simulink model "Model_Main_v4"  (R2025a)
settings: Solver=VariableStepAuto  StartTime=0.0  StopTime=10.0  RelTol=1e-3  AbsTol=1e-3
undefined symbols (not defined in the file): area_air, cp_air, eta_map, HC_min, HC_nom, rho_air, speed_bp_rpm, torque_bp_Nm, vel_air_nom
libraries: fl_lib x26, nesl_utility x14, SimscapeFluids_lib x5
(part 3 of 3)

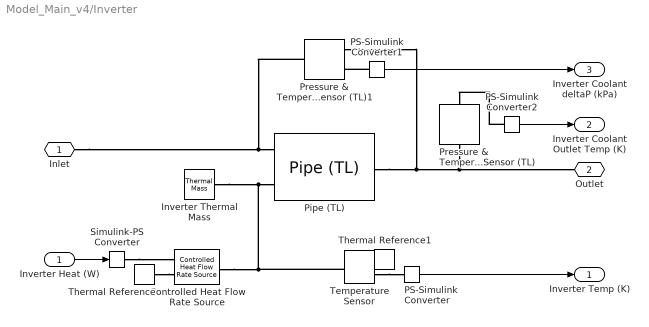
== system Model_Main_v4/Inverter ==
  Inverter Heat (W) : Inport
  Controlled Heat Flow Rate Source : fl_lib/Thermal/Thermal Sources/Controlled Heat Flow Rate Source
  Inverter Thermal Mass : fl_lib/Thermal/Thermal Elements/Thermal Mass  mass_type=foundation.enum.constant_variable.constant  mass=10 kg  sp_heat=900 J/(K*kg)  mass_min=1e-6 kg  num_ports=foundation.enum.numPorts2.one  m_specify=off  m_priority=High  m=1 kg  m_nominal_specify=off  m_nominal_value=1  m_nominal_unit=kg  T_specify=off  T_priority=High  T=300 K  T_nominal_specify=off  T_nominal_value=1  T_nominal_unit=K  Q_specify=off  Q_priority=None  Q=0 W  Q_nominal_specify=off  Q_nominal_value=1  Q_nominal_unit=W
  PS-Simulink Converter : nesl_utility/PS-Simulink Converter  PhysicalDomain=network_engine_domain  SubClassName=ps_output  LeftPortType=input  RightPortType=output  PseudoPeriodic=off  Frequencies=[]  VectorFormat=inherit  Unit=degC  AffineConversion=off
  PS-Simulink Converter1 : nesl_utility/PS-Simulink Converter  PhysicalDomain=network_engine_domain  SubClassName=ps_output  LeftPortType=input  RightPortType=output  PseudoPeriodic=off  Frequencies=[]  VectorFormat=inherit  Unit=kPa  AffineConversion=off
  PS-Simulink Converter2 : nesl_utility/PS-Simulink Converter  PhysicalDomain=network_engine_domain  SubClassName=ps_output  LeftPortType=input  RightPortType=output  PseudoPeriodic=off  Frequencies=[]  VectorFormat=inherit  Unit=degC  AffineConversion=off
  Pipe (TL) : fl_lib/Thermal Liquid/Elements/Pipe (TL)  length=3 m  area=5e-5 m^2  Dh=0.007 m  length_add=1 m  roughness=15e-6 m  Re_lam=2000  Re_tur=4000  shape_factor=64  Nu_lam=3.66  dynamic_compressibility=true  inertia=false  p0=0.101325 MPa  T0=293.15 K  mdot0=0 kg/s  p_nominal=0.101325 MPa  T_nominal=293.15 K
  Pressure & Temperature Sensor (TL) : fl_lib/Thermal Liquid/Sensors/Pressure & Temperature Sensor (TL)  reference=foundation.enum.MeasurementReference.absolute  pressure=false  pressure_spec=foundation.enum.PressureMeasementSpec.Absolute  temperature=true
      settings: InternalSimscapePortConfiguration="{\"Bottom\":[{\"id\":\"T\",\"label\":\"T\",\"type\":\"output\"}],\"Left\":[{\"id\":\"A\",\"label\":\"A\",\"type\":\"foundation.thermal_liquid.thermal_liquid\"}],\"Right\":[],\"Top\":[]}"
  Pressure & Temperature Sensor (TL)1 : fl_lib/Thermal Liquid/Sensors/Pressure & Temperature Sensor (TL)  reference=foundation.enum.MeasurementReference.difference  pressure=true  pressure_spec=foundation.enum.PressureMeasementSpec.Absolute  temperature=false
      settings: InternalSimscapePortConfiguration="{\"Bottom\":[],\"Left\":[{\"id\":\"A\",\"label\":\"A\",\"type\":\"foundation.thermal_liquid.thermal_liquid\"}],\"Right\":[{\"id\":\"B\",\"label\":\"B\",\"type\":\"foundation.thermal_liquid.thermal_liquid\"},{\"id\":\"P\",\"label\":\"P\",\"type\":\"output\"}],\"Top\":[]}"
  Simulink-PS Converter : nesl_utility/Simulink-PS Converter  PhysicalDomain=network_engine_domain  SubClassName=ps_input  LeftPortType=input  RightPortType=output  PseudoPeriodic=off  Frequencies=[]  NoiseDistribution=none  NoiseParameters=[]  Unit=W  AffineConversion=off  FilteringAndDerivatives=provide  SimscapeFilterOrder=1  InputFilterTimeConstant=0.001  UdotUserProvided=0
  Temperature Sensor : fl_lib/Thermal/Thermal Sensors/Temperature Sensor  temperature_measure=foundation.enum.MeasurementReference.difference
  Thermal Reference : fl_lib/Thermal/Thermal Elements/Thermal Reference
  Thermal Reference1 : fl_lib/Thermal/Thermal Elements/Thermal Reference
  Inlet : PMIOPort  Side=Left
  Outlet : PMIOPort  Port=2  Side=Right
  Inverter Temp (K) : Outport
  Inverter Coolant Outlet Temp (K) : Outport  Port=2
  Inverter Coolant deltaP (kPa) : Outport  Port=3
  wires:
  Inverter Heat (W)/1 -> Simulink-PS Converter/1
  PS-Simulink Converter/1 -> Inverter Temp (K)/1
  PS-Simulink Converter2/1 -> Inverter Coolant Outlet Temp (K)/1
  PS-Simulink Converter1/1 -> Inverter Coolant deltaP (kPa)/1
  connections:
  Inlet/RConn1 -- Pressure & Temperature Sensor (TL)1/LConn1 -- Pipe (TL)/LConn1
  Pipe (TL)/RConn1 -- Pressure & Temperature Sensor (TL)1/RConn1 -- Pressure & Temperature Sensor (TL)/LConn1 -- Outlet/RConn1
  Inverter Thermal Mass/LConn1 -- Temperature Sensor/LConn1 -- Controlled Heat Flow Rate Source/LConn1 -- Pipe (TL)/LConn2
  Thermal Reference/LConn1 -- Controlled Heat Flow Rate Source/RConn2
  Simulink-PS Converter/RConn1 -- Controlled Heat Flow Rate Source/RConn1
  Thermal Reference1/LConn1 -- Temperature Sensor/RConn1
  Temperature Sensor/RConn2 -- PS-Simulink Converter/LConn1
  PS-Simulink Converter1/LConn1 -- Pressure & Temperature Sensor (TL)1/RConn2
  PS-Simulink Converter2/LConn1 -- Pressure & Temperature Sensor (TL)/RConn1

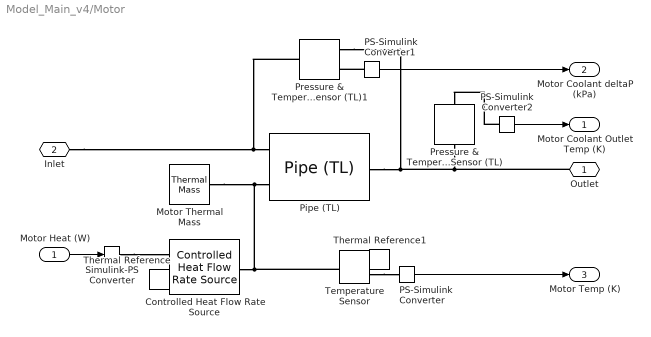
== system Model_Main_v4/Motor ==
  Motor Heat (W) : Inport
  Controlled Heat Flow Rate Source : fl_lib/Thermal/Thermal Sources/Controlled Heat Flow Rate Source
  Motor Thermal Mass : fl_lib/Thermal/Thermal Elements/Thermal Mass  mass_type=foundation.enum.constant_variable.constant  mass=24 kg  sp_heat=449 J/(K*kg)  mass_min=1e-6 kg  num_ports=foundation.enum.numPorts2.one  m_specify=off  m_priority=High  m=1 kg  m_nominal_specify=off  m_nominal_value=1  m_nominal_unit=kg  T_specify=off  T_priority=High  T=300 K  T_nominal_specify=off  T_nominal_value=1  T_nominal_unit=K  Q_specify=off  Q_priority=None  Q=0 W  Q_nominal_specify=off  Q_nominal_value=1  Q_nominal_unit=W
  PS-Simulink Converter : nesl_utility/PS-Simulink Converter  PhysicalDomain=network_engine_domain  SubClassName=ps_output  LeftPortType=input  RightPortType=output  PseudoPeriodic=off  Frequencies=[]  VectorFormat=inherit  Unit=degC  AffineConversion=off
  PS-Simulink Converter1 : nesl_utility/PS-Simulink Converter  PhysicalDomain=network_engine_domain  SubClassName=ps_output  LeftPortType=input  RightPortType=output  PseudoPeriodic=off  Frequencies=[]  VectorFormat=inherit  Unit=kPa  AffineConversion=off
  PS-Simulink Converter2 : nesl_utility/PS-Simulink Converter  PhysicalDomain=network_engine_domain  SubClassName=ps_output  LeftPortType=input  RightPortType=output  PseudoPeriodic=off  Frequencies=[]  VectorFormat=inherit  Unit=degC  AffineConversion=off
  Pipe (TL) : fl_lib/Thermal Liquid/Elements/Pipe (TL)  length=0.8 m  area=7.5e-6 m^2  Dh=0.023077 m  length_add=1 m  roughness=15e-6 m  Re_lam=2000  Re_tur=4000  shape_factor=64  Nu_lam=3.66  dynamic_compressibility=true  inertia=false  p0=0.101325 MPa  T0=293.15 K  mdot0=0 kg/s  p_nominal=0.101325 MPa  T_nominal=293.15 K
  Pressure & Temperature Sensor (TL) : fl_lib/Thermal Liquid/Sensors/Pressure & Temperature Sensor (TL)  reference=foundation.enum.MeasurementReference.absolute  pressure=false  pressure_spec=foundation.enum.PressureMeasementSpec.Absolute  temperature=true
      settings: InternalSimscapePortConfiguration="{\"Bottom\":[{\"id\":\"T\",\"label\":\"T\",\"type\":\"output\"}],\"Left\":[{\"id\":\"A\",\"label\":\"A\",\"type\":\"foundation.thermal_liquid.thermal_liquid\"}],\"Right\":[],\"Top\":[]}"
  Pressure & Temperature Sensor (TL)1 : fl_lib/Thermal Liquid/Sensors/Pressure & Temperature Sensor (TL)  reference=foundation.enum.MeasurementReference.difference  pressure=true  pressure_spec=foundation.enum.PressureMeasementSpec.Absolute  temperature=false
      settings: InternalSimscapePortConfiguration="{\"Bottom\":[],\"Left\":[{\"id\":\"A\",\"label\":\"A\",\"type\":\"foundation.thermal_liquid.thermal_liquid\"}],\"Right\":[{\"id\":\"B\",\"label\":\"B\",\"type\":\"foundation.thermal_liquid.thermal_liquid\"},{\"id\":\"P\",\"label\":\"P\",\"type\":\"output\"}],\"Top\":[]}"
  Simulink-PS Converter : nesl_utility/Simulink-PS Converter  PhysicalDomain=network_engine_domain  SubClassName=ps_input  LeftPortType=input  RightPortType=output  PseudoPeriodic=off  Frequencies=[]  NoiseDistribution=none  NoiseParameters=[]  Unit=W  AffineConversion=off  FilteringAndDerivatives=provide  SimscapeFilterOrder=1  InputFilterTimeConstant=0.001  UdotUserProvided=0
  Temperature Sensor : fl_lib/Thermal/Thermal Sensors/Temperature Sensor  temperature_measure=foundation.enum.MeasurementReference.difference
  Thermal Reference : fl_lib/Thermal/Thermal Elements/Thermal Reference
  Thermal Reference1 : fl_lib/Thermal/Thermal Elements/Thermal Reference
  Outlet : PMIOPort  Side=Left
  Inlet : PMIOPort  Port=2  Side=Right
  Motor Coolant Outlet Temp (K) : Outport
  Motor Coolant deltaP (kPa) : Outport  Port=2
  Motor Temp (K) : Outport  Port=3
  wires:
  Motor Heat (W)/1 -> Simulink-PS Converter/1
  PS-Simulink Converter/1 -> Motor Temp (K)/1
  PS-Simulink Converter2/1 -> Motor Coolant Outlet Temp (K)/1
  PS-Simulink Converter1/1 -> Motor Coolant deltaP (kPa)/1
  connections:
  Pipe (TL)/LConn1 -- Inlet/RConn1 -- Pressure & Temperature Sensor (TL)1/LConn1
  Pressure & Temperature Sensor (TL)1/RConn1 -- Pipe (TL)/RConn1 -- Pressure & Temperature Sensor (TL)/LConn1 -- Outlet/RConn1
  Motor Thermal Mass/LConn1 -- Temperature Sensor/LConn1 -- Controlled Heat Flow Rate Source/LConn1 -- Pipe (TL)/LConn2
  Thermal Reference/LConn1 -- Controlled Heat Flow Rate Source/RConn2
  Simulink-PS Converter/RConn1 -- Controlled Heat Flow Rate Source/RConn1
  Thermal Reference1/LConn1 -- Temperature Sensor/RConn1
  Temperature Sensor/RConn2 -- PS-Simulink Converter/LConn1
  PS-Simulink Converter1/LConn1 -- Pressure & Temperature Sensor (TL)1/RConn2
  PS-Simulink Converter2/LConn1 -- Pressure & Temperature Sensor (TL)/RConn1

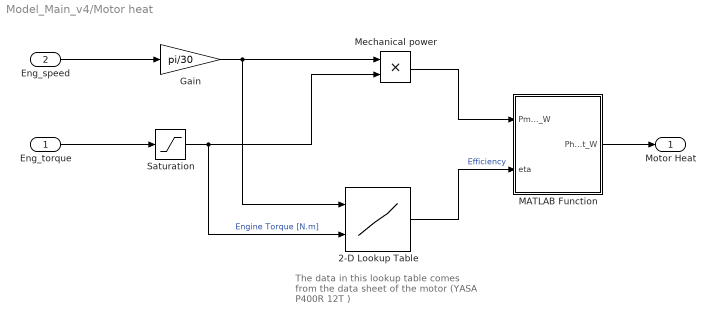
== system Model_Main_v4/Motor heat ==
  note: The data in this lookup table comes from the data sheet of the motor (YASA P400R 12T )
  Eng_torque : Inport
  Eng_speed : Inport  Port=2
  2-D Lookup Table : Lookup_n-D  BreakpointsForDimension1=torque_bp_Nm  BreakpointsForDimension2=speed_bp_rpm  Table=eta_map  InternalRulePriority=Speed  RndMeth=Simplest
      settings: InputPortMap=u0,u1
  Gain : Gain  Gain=pi/30
  MATLAB Function : MATLAB Function  TreatAsAtomicUnit=on
  Mechanical power : Product
  Saturation : Saturate  UpperLimit=inf  LowerLimit=0
  Motor Heat : Outport  VectorParamsAs1DForOutWhenUnconnected=off
  wires:
  Saturation/1 -> 2-D Lookup Table/2, Mechanical power/2  "Engine Torque [N.m]"
  Eng_torque/1 -> Saturation/1
  Gain/1 -> 2-D Lookup Table/1, Mechanical power/1
  Eng_speed/1 -> Gain/1
  2-D Lookup Table/1 -> MATLAB Function/2(eta)  "Efficiency"
  Mechanical power/1 -> MATLAB Function/1(Pmech_W)
  MATLAB Function/1(Pheat_W) -> Motor Heat/1

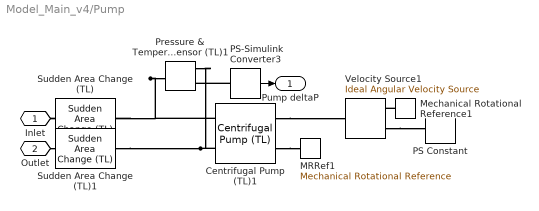
== system Model_Main_v4/Pump ==
  Centrifugal Pump (TL)1 : SimscapeFluids_lib/Thermal Liquid/Pumps & Motors/Centrifugal Pump (TL)  pump_parameterization=fluids.thermal_liquid.pumps_motors.enum.CentrifugalPumpParameterization.Table1D  capacity_ref_nominal=45 lpm  head_ref_nominal=40 m  power_ref_nominal=0.85 kW  head_ref_max=60 m  capacity_ref_max=80 lpm  omega_ref_analytic=1770 rpm  flow_rate_1D_TLU=|  head_1D_TLU=|  power_1D_TLU=[37 : 0.55 : 53]' kW  omega_ref_1D=3500 rpm  rho_ref_1D=820 kg/m^3  omega_threshold_factor=1e-2  flow_rate_2D_TLU=[16.67, 23.33, 30, 40, 53.33, 60] lpm  omega_2D_TLU=[2450, 2800, 3150, 3500] rpm  head_2D_TLU=[25, 32.7, 42.5, 50; 24, 31.7, 41, 49; 22.7, 30.5, 39, 47.5; 20, 28, 36, 45; 15.7, 24, 32, 40; 12.5, 21, 29.5, 37.5] m  power_2D_TLU=[.28, .38, .5, .6; .31, .41, .55, .68; .33, .44, .6, .75; .36, .48, .65, .83; .38, .53, .72, .93; .39, .55, .75, .97] kW  rho_ref_2D=998.21 kg/m^3  diameter_ratio=1  mech_orientation=fluids.thermal_liquid.pumps_motors.enum.CentrifugalPumpMechOrientation.Positive  area=0.01 m^2  operation_check=simscape.enum.assert.action.none
      flow_rate_1D_TLU=|
      | [0.047506301
      | 1.3064129510586207
      | 2.850356320364006
      | 4.2280281794317265
      | 5.3919244017967936
      | 6.484560628828113
      | 7.672209458087998
      | 9.02612871
      | 10.902614012716969
      | 12.589074110715908
      | 14.038005965117375
      | 15.84323018491505
      | 17.529692457563282
      | 19.311165157790786
      | 20.54631811351566
      | 21.852732151898927
      | 23.230405098291293
      | 24.845608462930425
      | 26.22327923
      | 27.577198486846402
      | 28.717341014992005
      | 30.02375287872598
      | 30.99762607128321
      | 32.161520118998986
      | 32.921616587528916
      | 33.56294675961082
      | 34.06175911567452
      | 34.465561044158946
      | 34.75059667619534
      | 35.01187643936299] lpm
      head_1D_TLU=|
      | [8.340175953079179
      |  8.252199346368963
      | 8.146627499
      |  8.014662488115148
      | 7.891495601
      |  7.750732869346819
      |  7.557184616491591
      |  7.310850439882696
      |  6.950146493324437
      |  6.6246334310850425
      |  6.316715408280447
      | 5.938416422
      |  5.5865099954465265
      |  5.225806451612903
      |  4.935483870967742
      |  4.627565445438508
      |  4.240468939728053
      |  3.7565977035030245
      |  3.263929350285237
      |  2.8328440378138744
      |  2.480938416422288
      |  2.0674481433857226
      |  1.7859234851825987
      |  1.4340170583417344
      |  1.2052783238922766
      |  0.9589437445587442
      |  0.7214070876672484
      |  0.4310845070220865
      |  0.19354785013059214
      | 0] m
      settings: InternalSimscapePortConfiguration="{\"Bottom\":[],\"Left\":[{\"id\":\"A\",\"label\":\"A\",\"type\":\"foundation.thermal_liquid.thermal_liquid\"},{\"id\":\"B\",\"label\":\"B\",\"type\":\"foundation.thermal_liquid.thermal_liquid\"}],\"Right\":[{\"id\":\"R\",\"label\":\"R\",\"type\":\"foundation.mechanical.rotational.rotational\"},{\"id\":\"C\",\"label\":\"C\",\"type\":\"foundation.mechanical.rotational.rotational\"}],\"Top\":[]}"
  MRRef1 : fl_lib/Mechanical/Rotational Elements/Mechanical Rotational Reference
  Mechanical Rotational Reference1 : fl_lib/Mechanical/Rotational Elements/Mechanical Rotational Reference
  PS Constant : fl_lib/Physical Signals/Sources/PS Constant  constant=3500 rpm
  PS-Simulink Converter3 : nesl_utility/PS-Simulink Converter  PhysicalDomain=network_engine_domain  SubClassName=ps_output  LeftPortType=input  RightPortType=output  PseudoPeriodic=off  Frequencies=[]  VectorFormat=1-D array  Unit=Pa  AffineConversion=on
  Pressure & Temperature Sensor (TL)1 : fl_lib/Thermal Liquid/Sensors/Pressure & Temperature Sensor (TL)  reference=foundation.enum.MeasurementReference.difference  pressure=true  pressure_spec=foundation.enum.PressureMeasementSpec.Absolute  temperature=false
      settings: InternalSimscapePortConfiguration="{\"Bottom\":[],\"Left\":[{\"id\":\"A\",\"label\":\"A\",\"type\":\"foundation.thermal_liquid.thermal_liquid\"}],\"Right\":[{\"id\":\"B\",\"label\":\"B\",\"type\":\"foundation.thermal_liquid.thermal_liquid\"},{\"id\":\"P\",\"label\":\"P\",\"type\":\"output\"}],\"Top\":[]}"
  Sudden Area Change (TL) : SimscapeFluids_lib/Thermal Liquid/Pipes & Fittings/Sudden Area Change (TL)  loss_spec=fluids.thermal_liquid.enum.area_change_loss_spec.empirical  area_A=0.02 m^2  area_B=0.01 m^2  K_c=1  K_e=1  Re_TLU=[10, 20, 30, 40, 50, 100, 200, 500, 1000, 2000]  loss_contraction_TLU=[5, 2.7, 1.8, 1.46, 1.3, .9, .65, .42, .3, .2]  loss_expansion_TLU=[3.1, 2.3, 1.65, 1.35, 1.15, .9, .75, .65, .9, .65]  Re_critical=150
      settings: InternalSimscapePortConfiguration="{\"Bottom\":[],\"Left\":[{\"id\":\"A\",\"label\":\"A\",\"type\":\"foundation.thermal_liquid.thermal_liquid\"}],\"Right\":[{\"id\":\"B\",\"label\":\"B\",\"type\":\"foundation.thermal_liquid.thermal_liquid\"}],\"Top\":[]}"
  Sudden Area Change (TL)1 : SimscapeFluids_lib/Thermal Liquid/Pipes & Fittings/Sudden Area Change (TL)  loss_spec=fluids.thermal_liquid.enum.area_change_loss_spec.empirical  area_A=0.02 m^2  area_B=0.01 m^2  K_c=1  K_e=1  Re_TLU=[10, 20, 30, 40, 50, 100, 200, 500, 1000, 2000]  loss_contraction_TLU=[5, 2.7, 1.8, 1.46, 1.3, .9, .65, .42, .3, .2]  loss_expansion_TLU=[3.1, 2.3, 1.65, 1.35, 1.15, .9, .75, .65, .9, .65]  Re_critical=150
      settings: InternalSimscapePortConfiguration="{\"Bottom\":[],\"Left\":[{\"id\":\"A\",\"label\":\"A\",\"type\":\"foundation.thermal_liquid.thermal_liquid\"}],\"Right\":[{\"id\":\"B\",\"label\":\"B\",\"type\":\"foundation.thermal_liquid.thermal_liquid\"}],\"Top\":[]}"
  Velocity Source1 : fl_lib/Mechanical/Mechanical Sources/Ideal Angular Velocity Source
  Inlet : PMIOPort  Side=Right
  Outlet : PMIOPort  Port=2  Side=Left
  Pump deltaP : Outport
  wires:
  PS-Simulink Converter3/1 -> Pump deltaP/1
  connections:
  Mechanical Rotational Reference1/LConn1 -- Velocity Source1/RConn2
  Centrifugal Pump (TL)1/RConn1 -- Velocity Source1/LConn1
  Outlet/RConn1 -- Sudden Area Change (TL)1/RConn1
  Pressure & Temperature Sensor (TL)1/LConn1 -- Sudden Area Change (TL)/LConn1 -- Centrifugal Pump (TL)1/LConn1
  Centrifugal Pump (TL)1/RConn2 -- MRRef1/LConn1
  PS-Simulink Converter3/LConn1 -- Pressure & Temperature Sensor (TL)1/RConn2
  Velocity Source1/RConn1 -- PS Constant/RConn1
  Inlet/RConn1 -- Sudden Area Change (TL)/RConn1
  Sudden Area Change (TL)1/LConn1 -- Pressure & Temperature Sensor (TL)1/RConn1 -- Centrifugal Pump (TL)1/LConn2

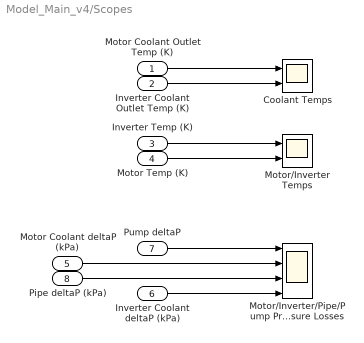
== system Model_Main_v4/Scopes ==
  Motor Coolant Outlet Temp (K) : Inport
  Inverter Coolant Outlet Temp (K) : Inport  Port=2
  Inverter Temp (K) : Inport  Port=3
  Motor Temp (K) : Inport  Port=4
  Motor Coolant deltaP (kPa) : Inport  Port=5
  Inverter Coolant deltaP (kPa) : Inport  Port=6
  Pump deltaP : Inport  Port=7
  Pipe deltaP (kPa) : Inport  Port=8
  Coolant Temps : Scope  NumInputPorts=2
      settings: ActiveDisplayYMinimum=291.78438285634167  ActiveDisplayYMaximum=301.8823145700498
  Motor/Inverter Temps : Scope  NumInputPorts=2
      settings: ActiveDisplayYMinimum=299.93626905750625  ActiveDisplayYMaximum=300.51975592912748
  Motor/Inverter/Pipe/Pump Pressure Losses : Scope  NumInputPorts=4
      settings: ActiveDisplayYMinimum=-75289.318426038168  ActiveDisplayYMaximum=28645.473693309257  DataLoggingVariableName=ScopeData2
  wires:
  Inverter Coolant Outlet Temp (K)/1 -> Coolant Temps/2
  Motor Coolant Outlet Temp (K)/1 -> Coolant Temps/1
  Motor Temp (K)/1 -> Motor/Inverter Temps/2
  Inverter Temp (K)/1 -> Motor/Inverter Temps/1
  Pipe deltaP (kPa)/1 -> Motor/Inverter/Pipe/Pump Pressure Losses/3
  Motor Coolant deltaP (kPa)/1 -> Motor/Inverter/Pipe/Pump Pressure Losses/2
  Inverter Coolant deltaP (kPa)/1 -> Motor/Inverter/Pipe/Pump Pressure Losses/4
  Pump deltaP/1 -> Motor/Inverter/Pipe/Pump Pressure Losses/1

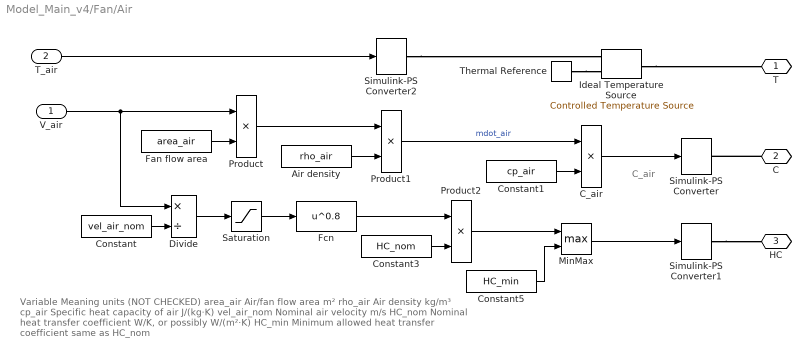
== system Model_Main_v4/Fan/Air ==
  note: Variable
      | Meaning
      | units (NOT CHECKED)
      |
      | area_air
      | Air/fan flow area
      | m²
      |
      | rho_air
      | Air density
      | kg/m³
      |
      | cp_air
      | Specific heat capacity of air
      | J/(kg·K)
      |
      | vel_air_nom
      | Nominal air velocity
      | m/s
      |
      | HC_nom
      | Nominal heat transfer coefficient
      | W/K, or possibly W/(m²·K)
      |
      | HC_min
      | Minimum allowed heat transfer coefficient
      | same as HC_nom
  note: C_air
  V_air : Inport
  T_air : Inport  Port=2
  Air density : Constant  Value=rho_air
  C_air : Product
  Constant : Constant  Value=vel_air_nom
  Constant1 : Constant  Value=cp_air
  Constant3 : Constant  Value=HC_nom
  Constant5 : Constant  Value=HC_min
  Divide : Product  Inputs=*/
  Fan flow area : Constant  Value=area_air
  Fcn : Fcn  Expr=u^0.8
  Ideal Temperature Source : fl_lib/Thermal/Thermal Sources/Controlled Temperature Source
  MinMax : MinMax  Function=max  Inputs=2
  Product : Product
  Product1 : Product
  Product2 : Product
  Saturation : Saturate  UpperLimit=inf  LowerLimit=0
  Simulink-PS Converter : nesl_utility/Simulink-PS Converter  PhysicalDomain=network_engine_domain  SubClassName=ps_input  LeftPortType=input  RightPortType=output  PseudoPeriodic=off  Frequencies=[]  NoiseDistribution=none  NoiseParameters=[]  Unit=W/K  AffineConversion=off  FilteringAndDerivatives=zero  SimscapeFilterOrder=1  InputFilterTimeConstant=1  UdotUserProvided=1
  Simulink-PS Converter1 : nesl_utility/Simulink-PS Converter  PhysicalDomain=network_engine_domain  SubClassName=ps_input  LeftPortType=input  RightPortType=output  PseudoPeriodic=off  Frequencies=[]  NoiseDistribution=none  NoiseParameters=[]  Unit=W/(m^2*K)  AffineConversion=off  FilteringAndDerivatives=zero  SimscapeFilterOrder=1  InputFilterTimeConstant=1  UdotUserProvided=1
  Simulink-PS Converter2 : nesl_utility/Simulink-PS Converter  PhysicalDomain=network_engine_domain  SubClassName=ps_input  LeftPortType=input  RightPortType=output  PseudoPeriodic=off  Frequencies=[]  NoiseDistribution=none  NoiseParameters=[]  Unit=K  AffineConversion=on  FilteringAndDerivatives=zero  SimscapeFilterOrder=1  InputFilterTimeConstant=1  UdotUserProvided=1
  Thermal Reference : fl_lib/Thermal/Thermal Elements/Thermal Reference
  T : PMIOPort  Side=Right
  C : PMIOPort  Port=2  Side=Right
  HC : PMIOPort  Port=3  Side=Right
  wires:
  V_air/1 -> Product/1, Divide/1
  Constant/1 -> Divide/2
  Constant3/1 -> Product2/2
  Divide/1 -> Saturation/1
  Fcn/1 -> Product2/1
  Product2/1 -> MinMax/1
  Constant5/1 -> MinMax/2
  MinMax/1 -> Simulink-PS Converter1/1
  T_air/1 -> Simulink-PS Converter2/1
  Constant1/1 -> C_air/2
  C_air/1 -> Simulink-PS Converter/1
  Product/1 -> Product1/1
  Air density/1 -> Product1/2
  Fan flow area/1 -> Product/2
  Product1/1 -> C_air/1  "mdot_air"
  Saturation/1 -> Fcn/1
  connections:
  C/RConn1 -- Simulink-PS Converter/RConn1
  Simulink-PS Converter1/RConn1 -- HC/RConn1
  Thermal Reference/LConn1 -- Ideal Temperature Source/RConn2
  Simulink-PS Converter2/RConn1 -- Ideal Temperature Source/RConn1
  Ideal Temperature Source/LConn1 -- T/RConn1

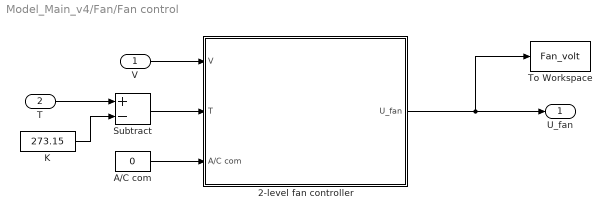
== system Model_Main_v4/Fan/Fan control ==
  V : Inport
  T : Inport  Port=2
  2-level fan controller : Subsystem
  A/C com : Constant  Value=0
  K : Constant  Value=273.15
  Subtract : Sum  Inputs=+-
  To Workspace : ToWorkspace  VariableName=Fan_volt  SampleTime=-1
  U_fan : Outport  VectorParamsAs1DForOutWhenUnconnected=off
  wires:
  K/1 -> Subtract/2
  T/1 -> Subtract/1
  A/C com/1 -> 2-level fan controller/3(A/C com)
  Subtract/1 -> 2-level fan controller/2(T)
  V/1 -> 2-level fan controller/1(V)
  2-level fan controller/1(U_fan) -> To Workspace/1, U_fan/1

== system Model_Main_v4/Fan/Fan unit ==
  Veh_speed : Inport
  U_fan : Inport  Port=2
  2D Lookup Table : Lookup_n-D  LookupTableObject=''  BreakpointsForDimension1=[0,40,90,110,150,180,198]  BreakpointsForDimension2=[0 14.4]  Table=[0,0.8,2.2,2.7,3.6,4.1,4.6; 1.5,2.3,3.2,3.5,4.3,4.8,5.1]'  InternalRulePriority=Speed  RndMeth=Simplest
      settings: InputPortMap=u0,u1
  Transfer Fcn : TransferFcn  Denominator=[10 1]
  V_air : Outport  VectorParamsAs1DForOutWhenUnconnected=off
  wires:
  Veh_speed/1 -> 2D Lookup Table/1
  2D Lookup Table/1 -> Transfer Fcn/1
  U_fan/1 -> 2D Lookup Table/2
  Transfer Fcn/1 -> V_air/1

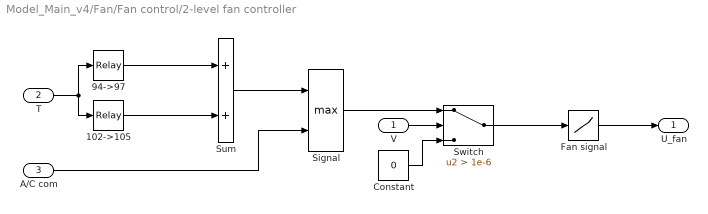
== system Model_Main_v4/Fan/Fan control/2-level fan controller ==
  V : Inport
  T : Inport  Port=2
  A/C com : Inport  Port=3
  102->105 : Relay  OnSwitchValue=T_level2(1)  OffSwitchValue=T_level2(2)
  94->97 : Relay  OnSwitchValue=T_level1(1)  OffSwitchValue=T_level1(2)
  Constant : Constant  Value=0
  Fan signal : Lookup  InputValues=[0, 1, 2]  Table=[0, 5, 14.4]
  Signal : MinMax  Function=max  Inputs=2  InputSameDT=on  SaturateOnIntegerOverflow=on
  Sum : Sum  Inputs=2  InputSameDT=on  SaturateOnIntegerOverflow=on  OutDataTypeStr=Inherit: Same as first input
  Switch : Switch  Criteria=u2 > Threshold  Threshold=1e-6  ZeroCross=off  SaturateOnIntegerOverflow=off  InputSameDT=off
  U_fan : Outport  VectorParamsAs1DForOutWhenUnconnected=off
  wires:
  Fan signal/1 -> U_fan/1
  T/1 -> 102->105/1, 94->97/1
  102->105/1 -> Sum/2
  94->97/1 -> Sum/1
  Sum/1 -> Signal/1
  Signal/1 -> Switch/1
  A/C com/1 -> Signal/2
  V/1 -> Switch/2
  Constant/1 -> Switch/3
  Switch/1 -> Fan signal/1

== matlab function Model_Main_v4/Motor heat/MATLAB Function ==
  data: Pheat_W output; Pmech_W input; eta input
function Pheat_W = heat_generation(Pmech_W, eta)

eta = max(eta, 0.01);

Pheat_W = Pmech_W * (1/eta - 1);

end
